simulink model "Parallel_R2017b"  (R2017b)
settings: Solver=ode4  StartTime=0  StopTime=1200  FixedStep=0.1  MaxStep=0.05  RelTol=1e-5
values from neighbouring files (symbols this model uses):
  Cd = 0.26    [Parallel_Initiate.m]
  Cr = 0.008    [Parallel_Initiate.m]
  Density = (85*19.6e6 + 15*32e6)/100    (= 21460000)    [Parallel_Initiate.m]
  Depletion = 0    [Parallel_Initiate.m]
  EMpower = EMpower_simulated(i)    [Batch_vary_rated_power.m]    (also in Parallel_Initiate.m = 50000)
  EtaICE = EtaICE_DIESEL    [Parallel_Initiate.m]
  EtaPE = 0.98    [Parallel_Initiate.m]
  grav = 9.81    [Parallel_Initiate.m]
  Hybrid = 1    [Parallel_Initiate.m]
  ICEpower = ICEpower_simulated(i)    [Batch_vary_rated_power.m]    (also in Parallel_Initiate.m = 65973)
  ksoc = max(Wbatt)/400/Tau_charge    [Parallel_Initiate.m]
  Mv = 1325 + 250    (= 1575)    [Parallel_Initiate.m]
  Number_of_gears = 5    [Parallel_Initiate.m]
  OnOffMax = SOC_batt_ref - eps    [Parallel_Initiate.m]
  OnOffMin = 30    [Parallel_Initiate.m]
  Paux = 600    [Parallel_Initiate.m]
  Pem_max = EMpower*Hybrid+2000*(1-Hybrid)    (= 50000)    [Parallel_Initiate.m]
  Pice_max = ICEpower*Hybrid+ICEconventional*(1-Hybrid)    (= 65973)    [Parallel_Initiate.m]
  rho_air = 1.225    [Parallel_Initiate.m]
  rw = 0.30    (= 0.3)    [Parallel_Initiate.m]
  SOC_batt_ref = 70    [Parallel_Initiate.m]
  StopAndGo = 0    [Parallel_Initiate.m]
  Tau_charge = 1    [Parallel_Initiate.m]
  Tem_max = TorqueEMmax*Hybrid+10*(1-Hybrid)    (= 400)    [Parallel_Initiate.m]
  Tice_max = Pice_max/(wice_max*row/(length(EtaICE)-1))    [Parallel_Initiate.m]
  utvx_max = wice_max/((vmax/5)/rw)    (= 15.9043128088)    [Parallel_Initiate.m]
  utvx_min = wice_max/(vmax/rw)/1.3    (= 2.4468173552)    [Parallel_Initiate.m]
  Utvx_vect = zeros(1,Number_of_gears+1)    [Parallel_Initiate.m]
  vmax = 160/3.6    (= 44.4444444444)    [Parallel_Initiate.m]
  Wbatt = 100*3600*13    (= 4680000)    [Parallel_Initiate.m]
  wice_max = 4500*2*pi/60    (= 471.238898038)    [Parallel_Initiate.m]
  wice_min = 800*2*pi/60    (= 83.7758040957)    [Parallel_Initiate.m]
undefined symbols (not defined in the file or in its folder): Av, EtaBATT, EtaEM, FuelConsICE, Pbatt, Pice_max_parallel, PtoT, sfunxy, Tem, Tice, Tlim_ice, Wem, Wice
libraries: simulink_need_slupdate x1
settings Model: ExtModeTrigMode=oneshot  ExtModeArmWhenConnect=off  Creator=matsl  LastModifiedBy=leksell
settings DataIOCC: SaveFormat=Array  SignalLoggingSaveFormat=ModelDataLogs  SignalLoggingName=sigsOut
settings OptimizationCC: BlockReduction=off  BooleanDataType=off  ExpressionDepthLimit=2147483647  InitFltsAndDblsToZero=on  LifeSpan=inf
settings DebuggingCC: ConsistencyChecking=warning  SaveWithParameterizedLinksMsg=none  UnderspecifiedInitializationDetection=Classic  MergeDetectMultiDrivingBlocksExec=none  SignalResolutionControl=TryResolveAllWithWarning  MultiTaskDSMMsg=warning  MultiTaskCondExecSysMsg=none  UnnecessaryDatatypeConvMsg=warning  FcnCallInpInsideContextMsg=warning  UnconnectedInputMsg=none  UnconnectedOutputMsg=none  UnconnectedLineMsg=none  AllowSymbolicDim=off  StateNameClashWarn=warning  SFUnexpectedBacktrackingDiag=warning  SFNoUnconditionalDefaultTransitionDiag=warning  SFExecutionAtInitializationDiag=none
settings HardwareCC: ProdBitPerPointer=32  ProdBitPerSizeT=32  ProdBitPerPtrDiffT=32  ProdLargestAtomicFloat=None  ProdIntDivRoundTo=Undefined  ProdEndianess=Unspecified  ProdWordSize=32  ProdHWDeviceType=32-bit Generic  TargetBitPerPointer=64  TargetBitPerSizeT=64  TargetBitPerPtrDiffT=64  TargetLongLongMode=on  TargetIntDivRoundTo=Zero  TargetEndianess=LittleEndian  TargetWordSize=64  TargetHWDeviceType=MATLAB Host  ProdEqTarget=off
settings ModelReferenceCC: PropagateSignalLabelsOutOfModel=off
settings CodeAppCC: StateflowObjectComments=on
settings GRTTargetCC: TargetFcnLib=ansi_tfl_tmw.mat  TargetLangStandard=C89/C90 (ANSI)  GeneratePreprocessorConditionals=Disable all  CombineOutputUpdateFcns=off  GRTInterface=on
settings ConfigComp: CovMetricSettings=dw  CovHtmlReporting=on  CovSaveCumulativeToWorkspaceVar=on  CovSaveSingleToWorkspaceVar=on  CovExternalEMLEnable=off

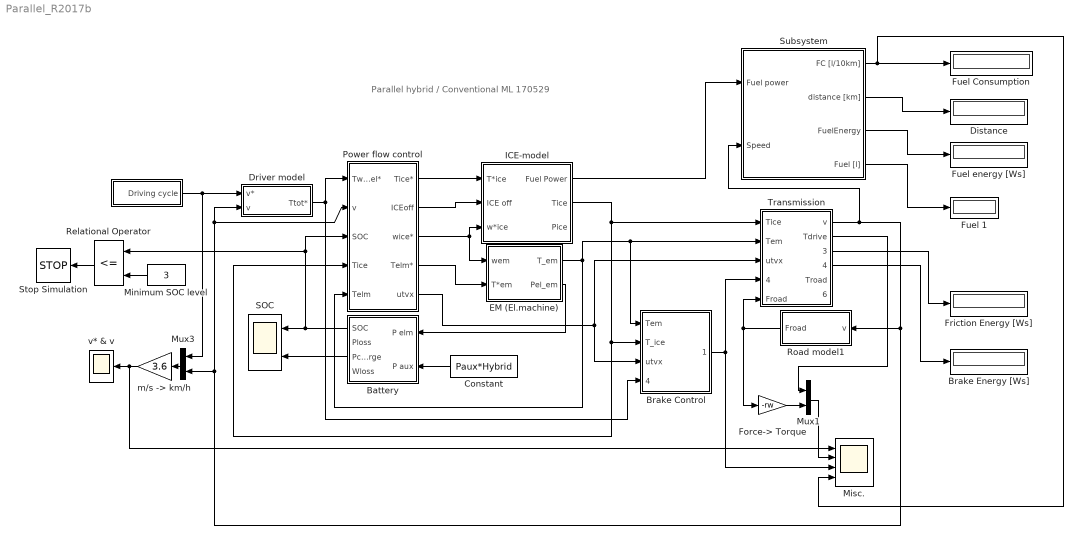
== system Parallel_R2017b ==
  note: Parallel hybrid / Conventional
      | ML 170529
  " " : Subsystem  mask{Cycle=us06}
      mask prompts: Cycle "Driving cycle"
      mask TypeOptions Cycle: nedc | us06 | IdealMotion
  Battery : Subsystem
  Brake Control : Subsystem
  Brake Energy [Ws] : Display
  Constant : Constant  Value=Paux*Hybrid
  Distance : Display
  "Driver model " : Subsystem  mask{Mv=Mv, rw=rw, T_max=(ICEpower+EMpower)/(vmax/rw)*utvx_min}
      mask prompts: Mv "Vehicle Mass"; rw "Wheel Radius"; T_max "Max Wheel Torque"
      mask init:
      | Ti = 3 + 7*(Mv-1000)/9000;
      | Kv=4*Mv/Ti;
  EM (El.machine) : Subsystem
  Force-> Torque : Gain  Gain=-rw  SaturateOnIntegerOverflow=on  OutDataTypeStr=Inherit: Same as input  ParamDataTypeStr=Inherit: Same as input
  Friction Energy [Ws] : Display
  Fuel 1 : Display
  Fuel Consumption : Display
  Fuel energy [Ws] : Display
  ICE-model : Subsystem
  Minimum SOC level : Constant  Value=3
  Misc. : Scope  NumInputPorts=4
  Mux1 : Mux  Inputs=2
  Mux3 : Mux  Inputs=2
  Power flow control : Subsystem
  Relational Operator : RelationalOperator  Operator=<=  OutDataTypeStr=boolean  RndMeth=Nearest
  Road model1 : Subsystem
  SOC : Scope  NumInputPorts=2
  Stop Simulation : Stop
  Subsystem : Subsystem
  Transmission : Subsystem
  "m/s -> km/h" : Gain  Gain=3.6  SaturateOnIntegerOverflow=on  OutDataTypeStr=Inherit: Same as input  ParamDataTypeStr=Inherit: Same as input
  v* & v : Scope
  wires:
  Power flow control/3(wice*) -> EM (El.machine)/1(wem), ICE-model/3(w*ice)
  Constant/1 -> Battery/2(P aux)
  " "/1(Driving cycle) -> Mux3/1, "Driver model "/1(v*)
  "Driver model "/1(Ttot*) -> Brake Control/4(T*_wheel), Power flow control/1(Twheel*)
  Mux3/1 -> "m/s -> km/h"/1
  Power flow control/5(utvx) -> Transmission/3(utvx), Brake Control/3(utvx)
  Power flow control/4(Telm*) -> EM (El.machine)/2(T*em)
  Power flow control/1(Tice*) -> ICE-model/1(T*ice)
  Transmission/1(v) -> "Driver model "/2(v), Power flow control/2(v), Mux3/2, Road model1/1("v "), Subsystem/2(Speed)
  Road model1/1(Froad) -> Transmission/5(Froad), Force-> Torque/1
  EM (El.machine)/1(T_em) -> Transmission/2(Tem), Brake Control/1(Tem), Power flow control/5(Telm)
  EM (El.machine)/2(Pel_em) -> Battery/1(P elm)
  "m/s -> km/h"/1 -> v* & v/1, Misc./1
  Transmission/3(Wfriction) -> Friction Energy [Ws]/1
  Transmission/4(Wbrake) -> Brake Energy [Ws]/1
  Subsystem/1(FC [l/10km]) -> Misc./4, Fuel Consumption/1
  Brake Control/1(T_brake) -> Transmission/4(Tbrake), Misc./3
  Power flow control/2(ICEoff) -> ICE-model/2(ICE off)
  Battery/3(Pcharge) -> SOC/2
  ICE-model/2(Tice) -> Transmission/1(Tice), Power flow control/4(Tice), Brake Control/2(T_ice)
  ICE-model/1(Fuel Power) -> Subsystem/1(Fuel power)
  Subsystem/3(FuelEnergy) -> Fuel energy [Ws]/1
  Force-> Torque/1 -> Mux1/2
  Mux1/1 -> Misc./2
  Transmission/2(Tdrive) -> Mux1/1
  Subsystem/2(distance [km]) -> Distance/1
  Subsystem/4(Fuel [l]) -> Fuel 1/1
  Relational Operator/1 -> Stop Simulation/1
  Minimum SOC level/1 -> Relational Operator/2
  Battery/1(SOC) -> Power flow control/3(SOC), Relational Operator/1, SOC/1

== system Parallel_R2017b/  ==
  Constant : Constant  Value=Cycle
  Multiport Switch : MultiPortSwitch  SaturateOnIntegerOverflow=on  InputSameDT=on
  v-buss1 : FromWorkspace  VariableName=us06  SampleTime=.1
  v-buss2 : FromWorkspace  VariableName=IdealMotion  SampleTime=.1
  v-buss8 : FromWorkspace  VariableName=nedc  SampleTime=.1
  Driving cycle : Outport
  wires:
  v-buss8/1 -> Multiport Switch/2
  Constant/1 -> Multiport Switch/1
  v-buss1/1 -> Multiport Switch/3
  v-buss2/1 -> Multiport Switch/4
  Multiport Switch/1 -> Driving cycle/1

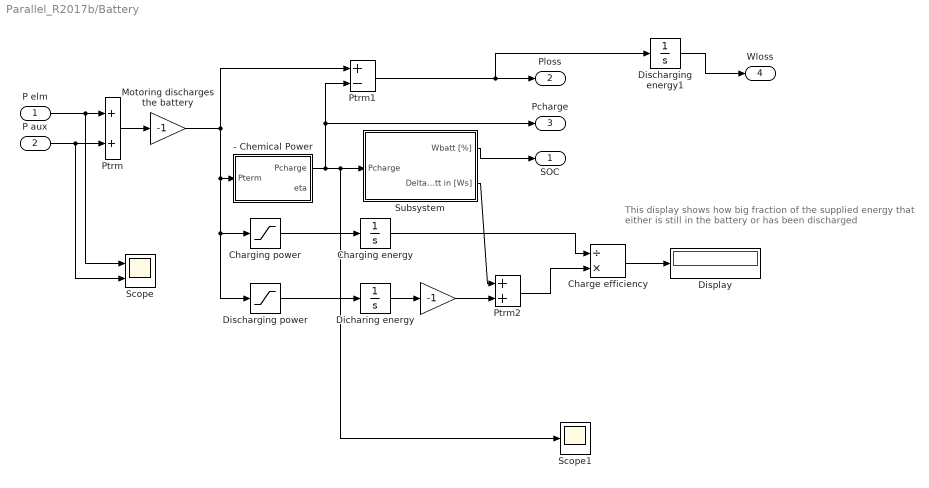
== system Parallel_R2017b/Battery ==
  note: This display shows how big fraction of the supplied energy
      | that either is still in the battery or has been discharged
  P elm : Inport
  P aux : Inport  Port=2
  " " : Gain  Gain=-1  SaturateOnIntegerOverflow=on  OutDataTypeStr=Inherit: Same as input  ParamDataTypeStr=Inherit: Same as input
  - Chemical Power : Subsystem
  Charge efficiency : Product  Inputs=/*  SaturateOnIntegerOverflow=on  OutDataTypeStr=Inherit: Same as first input
  Charging energy : Integrator  InitialCondition=1  LimitOutput=on  LowerSaturationLimit=1
  Charging power : Saturate  UpperLimit=inf  LowerLimit=0
  Dicharing energy : Integrator  InitialCondition=-1  LimitOutput=on  UpperSaturationLimit=-1
  Discharging energy1 : Integrator  UpperSaturationLimit=-1
  Discharging power : Saturate  UpperLimit=0  LowerLimit=-inf
  Display : Display
  Motoring discharges the battery : Gain  Gain=-1  SaturateOnIntegerOverflow=on  OutDataTypeStr=Inherit: Same as input  ParamDataTypeStr=Inherit: Same as input
  Ptrm : Sum  SaturateOnIntegerOverflow=on  InputSameDT=on  OutDataTypeStr=Inherit: Same as first input
  Ptrm1 : Sum  Inputs=+-  SaturateOnIntegerOverflow=on  InputSameDT=on  OutDataTypeStr=Inherit: Same as first input
  Ptrm2 : Sum  SaturateOnIntegerOverflow=on  InputSameDT=on  OutDataTypeStr=Inherit: Same as first input
  Scope : Scope  NumInputPorts=2
  Scope1 : Scope
  Subsystem : Subsystem
  SOC : Outport  InitialOutput=0
  Ploss : Outport  Port=2  InitialOutput=0
  Pcharge : Outport  Port=3  InitialOutput=0
  Wloss : Outport  Port=4  InitialOutput=0
  wires:
  P elm/1 -> Ptrm/1, Scope/1
  Ptrm/1 -> Motoring discharges the battery/1
  Subsystem/1(Wbatt [%]) -> SOC/1
  - Chemical Power/1(Pcharge) -> Ptrm1/2, Pcharge/1, Subsystem/1("Pcharge "), Scope1/1
  Ptrm1/1 -> Ploss/1, Discharging energy1/1
  Motoring discharges the battery/1 -> Ptrm1/1, Charging power/1, Discharging power/1, - Chemical Power/1(Pterm)
  Charge efficiency/1 -> Display/1
  Charging power/1 -> Charging energy/1
  Discharging power/1 -> Dicharing energy/1
  Dicharing energy/1 -> " "/1
  Subsystem/2(DeltaWbatt in [Ws]) -> Ptrm2/1
  " "/1 -> Ptrm2/2
  Ptrm2/1 -> Charge efficiency/2
  Charging energy/1 -> Charge efficiency/1
  P aux/1 -> Ptrm/2, Scope/2
  Discharging energy1/1 -> Wloss/1

== system Parallel_R2017b/Brake Control ==
  note: If the drive train is not able
      | to supply the braking force, then
      | the friction brakes are used.
  Tem : Inport
  T_ice : Inport  Port=2
  utvx : Inport  Port=3
  T*_wheel : Inport  Port=4
  -> wheel torque : Product  SaturateOnIntegerOverflow=on  InputSameDT=on  OutDataTypeStr=Inherit: Same as first input
  Only negative brake torque : Saturate  UpperLimit=0  LowerLimit=-inf
  Sum1 : Sum  Inputs=-+  SaturateOnIntegerOverflow=on  InputSameDT=on  OutDataTypeStr=Inherit: Same as first input
  Sum2 : Sum  SaturateOnIntegerOverflow=on  InputSameDT=on  OutDataTypeStr=Inherit: Same as first input
  T_brake : Outport  InitialOutput=0
  wires:
  Tem/1 -> Sum2/1
  T_ice/1 -> Sum2/2
  Sum2/1 -> -> wheel torque/1
  utvx/1 -> -> wheel torque/2
  -> wheel torque/1 -> Sum1/1
  T*_wheel/1 -> Sum1/2
  Sum1/1 -> Only negative brake torque/1
  Only negative brake torque/1 -> T_brake/1

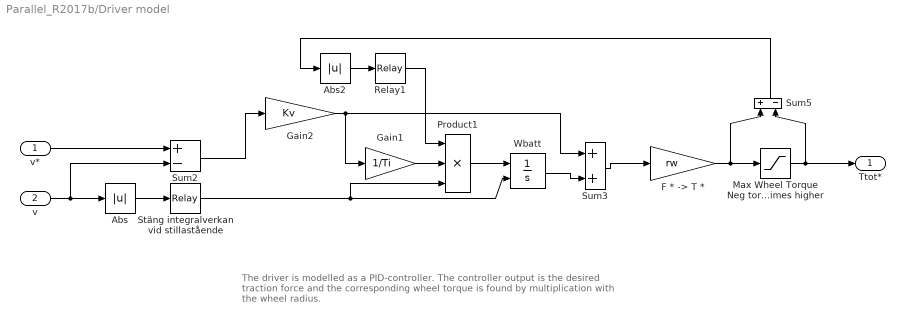
== system Parallel_R2017b/Driver model  ==
  note: The driver is modelled as a PID-controller.
      | The controller output is the desired traction force and the
      | corresponding wheel torque is found by multiplication with the wheel radius.
  v* : Inport
  v : Inport  Port=2
  Abs : Abs  SaturateOnIntegerOverflow=on
  Abs2 : Abs  SaturateOnIntegerOverflow=on
  "F * -> T *" : Gain  Gain=rw  SaturateOnIntegerOverflow=on  OutDataTypeStr=Inherit: Same as input  ParamDataTypeStr=Inherit: Same as input
  Gain1 : Gain  Gain=1/Ti  SaturateOnIntegerOverflow=on  OutDataTypeStr=Inherit: Same as input  ParamDataTypeStr=Inherit: Same as input
  Gain2 : Gain  Gain=Kv  SaturateOnIntegerOverflow=on  OutDataTypeStr=Inherit: Same as input  ParamDataTypeStr=Inherit: Same as input
  Max Wheel Torque Neg torque 5 times higher : Saturate  UpperLimit=T_max  LowerLimit=-T_max*5
  Product1 : Product  Inputs=3  SaturateOnIntegerOverflow=on  InputSameDT=on  OutDataTypeStr=Inherit: Same as first input
  Relay1 : Relay  OnOutputValue=0  OffOutputValue=1
  Stäng integralverkan vid stillastående : Relay  OnSwitchValue=0.3  OffSwitchValue=0.3-eps
  Sum2 : Sum  Inputs=+-  SaturateOnIntegerOverflow=on  InputSameDT=on  OutDataTypeStr=Inherit: Same as first input
  Sum3 : Sum  SaturateOnIntegerOverflow=on  InputSameDT=on  OutDataTypeStr=Inherit: Same as first input
  Sum5 : Sum  Inputs=+-  SaturateOnIntegerOverflow=on  InputSameDT=on  OutDataTypeStr=Inherit: Same as first input
  Wbatt : Integrator  ExternalReset=falling  LimitOutput=on  UpperSaturationLimit=1000  LowerSaturationLimit=-10000
  Ttot* : Outport  InitialOutput=0
  wires:
  Sum5/1 -> Abs2/1
  Max Wheel Torque Neg torque 5 times higher/1 -> Sum5/2, Ttot*/1
  Relay1/1 -> Product1/1
  Abs2/1 -> Relay1/1
  Gain1/1 -> Product1/2
  Abs/1 -> Stäng integralverkan vid stillastående/1
  Product1/1 -> Wbatt/1
  Sum3/1 -> "F * -> T *"/1
  Wbatt/1 -> Sum3/2
  "F * -> T *"/1 -> Sum5/1, Max Wheel Torque Neg torque 5 times higher/1
  Gain2/1 -> Gain1/1, Sum3/1
  Stäng integralverkan vid stillastående/1 -> Product1/3, Wbatt/2
  Sum2/1 -> Gain2/1
  v*/1 -> Sum2/1
  v/1 -> Abs/1, Sum2/2

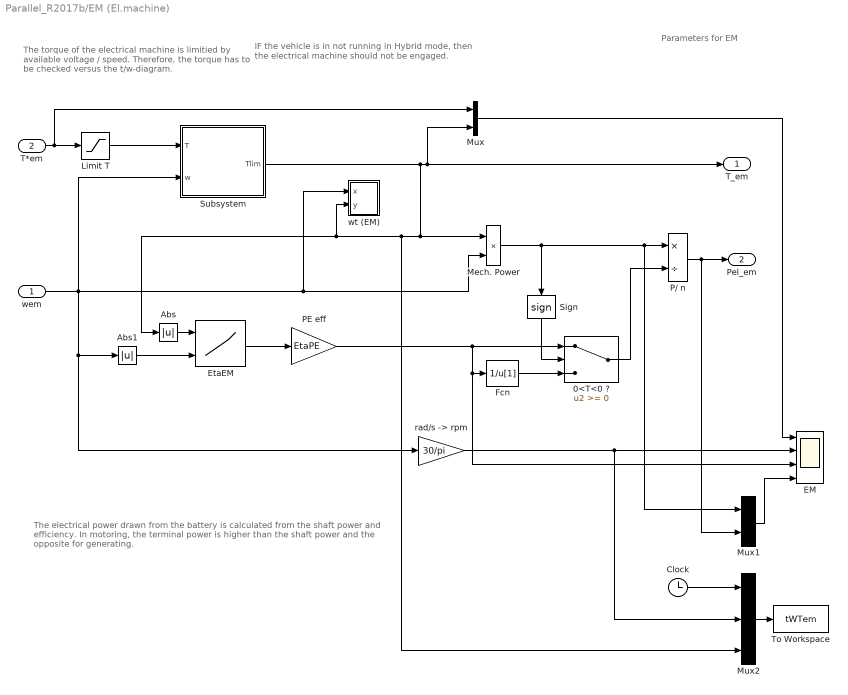
== system Parallel_R2017b/EM (El.machine) ==
  note: The torque of the electrical machine is
      | limitied by available voltage / speed. Therefore, the
      | torque has to be checked versus the t/w-diagram.
  note: IF the vehicle is in not running in Hybrid mode, then
      | the electrical machine should not be engaged.
  note: The electrical power drawn from the battery is calculated from the shaft power and
      | efficiency. In motoring, the terminal power is higher than the shaft power and
      | the opposite for  generating.
  note: Parameters for EM
  wem : Inport
  T*em : Inport  Port=2
  0<T<0 ? : Switch  SaturateOnIntegerOverflow=on  InputSameDT=on
  Abs : Abs  SaturateOnIntegerOverflow=on
  Abs1 : Abs  SaturateOnIntegerOverflow=on
  Clock : Clock
  "EM " : Scope  NumInputPorts=4
  EtaEM : Lookup2D  RowIndex=Tem  ColumnIndex=Wem  Table=EtaEM  LookUpMeth=Interpolation-Use End Values  SaturateOnIntegerOverflow=on
  Fcn : Fcn  Expr=1/u[1]
  Limit T : Saturate  UpperLimit=Tem_max  LowerLimit=-Tem_max
  Mech. Power : Product  SaturateOnIntegerOverflow=on  OutDataTypeStr=Inherit: Same as first input
  Mux : Mux  Inputs=2
  Mux1 : Mux  Inputs=2
  Mux2 : Mux  Inputs=3
  P/ n : Product  Inputs=*/  SaturateOnIntegerOverflow=on  InputSameDT=on  OutDataTypeStr=Inherit: Same as first input
  PE eff : Gain  Gain=EtaPE  SaturateOnIntegerOverflow=on  OutDataTypeStr=Inherit: Same as input  ParamDataTypeStr=Inherit: Same as input
  Sign : Signum
  Subsystem : Subsystem  mask{Tmax=Tem_max, Pmax=Pem_max}
      mask prompts: Tmax "Max Torque"; Pmax "Max Power"
      mask Display:
      | plot(-120,-120,120,120)
      | plot([-110 110],[0 0],[0 0],[-110 110])
      | plot([-20 20],[90 90],[-20 20],[-90 -90])
      | 
      | plot([-100 :-20],-90*20./[-100:-20])
      | plot([-100 :-20],90*20./[-100:-20])
      | plot([20:100],-90*20./[20:100])
      | plot([20:100],90*20./[20:100])
  To Workspace : ToWorkspace  VariableName=tWTem  SampleTime=-1
  "rad/s -> rpm" : Gain  Gain=30/pi  SaturateOnIntegerOverflow=on  OutDataTypeStr=Inherit: Same as input  ParamDataTypeStr=Inherit: Same as input
  wt (EM) : Subsystem  AncestorBlock=simulink/Sinks/XY Graph  LoadFcn=sfunxy([],[],[],'LoadBlock')  StartFcn=sfunxy([],[],[],'Start')  StopFcn=sfunxy([],[],[],'Stop')  TreatAsAtomicUnit=on  SimViewingDevice=on  mask(XY scope.){xmin=-max(Wem)*1.2, xmax=max(Wem)*1.2, ymin=-max(Tem)*1.2, ymax=max(Tem)*1.2, st=1}
      mask prompts: xmin "x-min:"; xmax "x-max:"; ymin "y-min:"; ymax "y-max:"; st "Sample time:"
      mask help: Plots second input (Y) against first input (X) at each time step to create an X-Y plot. Ignores data outside the ranges specified by x-min, x-max, y-min, y-max.
      settings: CopyFcn=sfunxy([],[],[],'CopyBlock')  DeleteFcn=sfunxy([],[],[],'DeleteBlock')  NameChangeFcn=sfunxy([],[],[],'NameChange')
      mask Help: This block can be used to explore limit cycles. Look at the m-file sfunxy.m to see how it works.
      mask Display: plot([.05 .95 .95 .05 .05],[.45 .45 .95 .95 .45], 0.5+cos(0:0.1:2*pi)*0.3,0.7+sin(0:0.1:2*pi)*0.2)
  T_em : Outport  InitialOutput=0
  Pel_em : Outport  Port=2  InitialOutput=0
  wires:
  EtaEM/1 -> PE eff/1
  Sign/1 -> 0<T<0 ?/2
  P/ n/1 -> Mux1/2, Pel_em/1
  T*em/1 -> Limit T/1, Mux/1
  Fcn/1 -> 0<T<0 ?/3
  0<T<0 ?/1 -> P/ n/2
  Abs/1 -> EtaEM/1
  Limit T/1 -> Subsystem/1(T)
  PE eff/1 -> "EM "/3, Fcn/1, 0<T<0 ?/1
  Mux/1 -> "EM "/1
  Mux1/1 -> "EM "/4
  Mech. Power/1 -> Sign/1, Mux1/1, P/ n/1
  Abs1/1 -> EtaEM/2
  wem/1 -> "rad/s -> rpm"/1, Abs1/1, wt (EM)/1(x), Mech. Power/2, Subsystem/2(w)
  Subsystem/1(Tlim) -> T_em/1, Mux/2, Mech. Power/1, wt (EM)/2(y), Abs/1, Mux2/3
  Clock/1 -> Mux2/1
  Mux2/1 -> To Workspace/1
  "rad/s -> rpm"/1 -> Mux2/2, "EM "/2

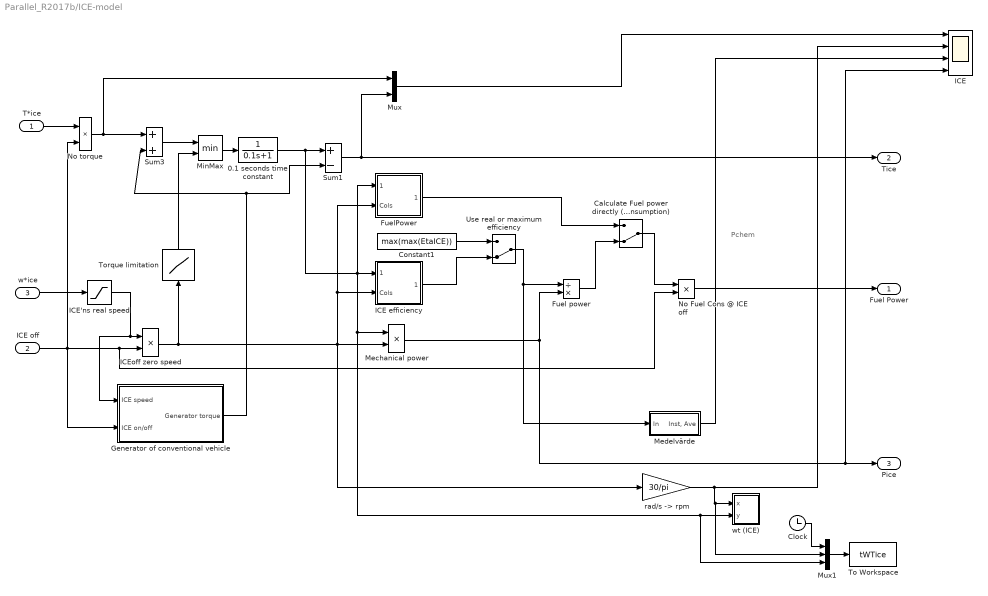
== system Parallel_R2017b/ICE-model ==
  note: Pchem
  T*ice : Inport
  ICE off : Inport  Port=2
  w*ice : Inport  Port=3
  0.1 seconds time constant : TransferFcn  Denominator=[0.1 1]
  Calculate Fuel power directly (w/o idle consumption) : ManualSwitch  CurrentSetting=0
  Clock : Clock
  Constant1 : Constant  Value=max(max(EtaICE))
  Fuel power : Product  Inputs=/*  SaturateOnIntegerOverflow=on  InputSameDT=on  OutDataTypeStr=Inherit: Same as first input
  FuelPower : Subsystem  mask(Lookup Table (2-D)){x=Tice, y=Wice, t=FuelConsICE}
      mask prompts: x "Row:"; y "Column:"; t "Table:"
      mask help: Performs 2-D linear interpolation of input values using the specified input/output table. Extrapolation is performed outside the table boundaries. The first dimension corresponds to the top (or left) input port.
      mask init:
      | [r,c]=size(t);
      | xt=reshape(x,prod(size(x)),1);
      | xi=xt(:,ones(1,c));
      | minx=min(x); maxx=max(x);
      | mint=min(min(t)); maxt=max(max(t));
      mask Display: plot(double(xi),double(t),double([minx maxx]),double([mint mint]),double([minx minx]),double([mint maxt]))
  Generator of conventional vehicle : Subsystem
  ICE : Scope  NumInputPorts=4
  ICE efficiency : Subsystem  mask(Lookup Table (2-D)){x=Tice, y=Wice, t=EtaICE}
      mask prompts: x "Row:"; y "Column:"; t "Table:"
      mask help: Performs 2-D linear interpolation of input values using the specified input/output table. Extrapolation is performed outside the table boundaries. The first dimension corresponds to the top (or left) input port.
      mask init:
      | [r,c]=size(t);
      | xt=reshape(x,prod(size(x)),1);
      | xi=xt(:,ones(1,c));
      | minx=min(x); maxx=max(x);
      | mint=min(min(t)); maxt=max(max(t));
      mask Display: plot(double(xi),double(t),double([minx maxx]),double([mint mint]),double([minx minx]),double([mint maxt]))
  ICE'ns real speed : Saturate  UpperLimit=wice_max  LowerLimit=wice_min
  ICEoff zero speed : Product  SaturateOnIntegerOverflow=on  InputSameDT=on  OutDataTypeStr=Inherit: Same as first input
  Mechanical power : Product  SaturateOnIntegerOverflow=on  InputSameDT=on  OutDataTypeStr=Inherit: Same as first input
  Medelvärde : Subsystem
  MinMax : MinMax  Inputs=2  SaturateOnIntegerOverflow=on  InputSameDT=on
  Mux : Mux  Inputs=2
  Mux1 : Mux  Inputs=3
  No Fuel Cons @ ICE off : Product  Inputs=**  SaturateOnIntegerOverflow=on  InputSameDT=on  OutDataTypeStr=Inherit: Same as first input
  No torque : Product  SaturateOnIntegerOverflow=on  OutDataTypeStr=Inherit: Same as first input
  Sum1 : Sum  Inputs=+-  SaturateOnIntegerOverflow=on
  Sum3 : Sum  SaturateOnIntegerOverflow=on
  To Workspace : ToWorkspace  VariableName=tWTice  SampleTime=-1
  Torque limitation : Lookup  InputValues=Wice  Table=Tlim_ice  SaturateOnIntegerOverflow=on
  Use real or maximum efficiency : ManualSwitch  CurrentSetting=0
  "rad/s -> rpm" : Gain  Gain=30/pi  SaturateOnIntegerOverflow=on  OutDataTypeStr=Inherit: Same as input  ParamDataTypeStr=Inherit: Same as input
  wt (ICE) : Subsystem  AncestorBlock=simulink/Sinks/XY Graph  LoadFcn=sfunxy([],[],[],'LoadBlock')  StartFcn=sfunxy([],[],[],'Start')  StopFcn=sfunxy([],[],[],'Stop')  TreatAsAtomicUnit=on  SimViewingDevice=on  mask(XY scope.){xmin=0, xmax=max(Wice)*30/pi*1.2, ymin=-max(Tice)*0.2, ymax=max(Tice)*1.2, st=1}
      mask prompts: xmin "x-min:"; xmax "x-max:"; ymin "y-min:"; ymax "y-max:"; st "Sample time:"
      mask help: Plots second input (Y) against first input (X) at each time step to create an X-Y plot. Ignores data outside the ranges specified by x-min, x-max, y-min, y-max.
      settings: CopyFcn=sfunxy([],[],[],'CopyBlock')  DeleteFcn=sfunxy([],[],[],'DeleteBlock')  NameChangeFcn=sfunxy([],[],[],'NameChange')
      mask Help: This block can be used to explore limit cycles. Look at the m-file sfunxy.m to see how it works.
      mask Display: plot([.05 .95 .95 .05 .05],[.45 .45 .95 .95 .45], 0.5+cos(0:0.1:2*pi)*0.3,0.7+sin(0:0.1:2*pi)*0.2)
  Fuel Power : Outport  InitialOutput=0
  Tice : Outport  Port=2  InitialOutput=0
  Pice : Outport  Port=3  InitialOutput=0
  wires:
  Mux/1 -> ICE/1
  MinMax/1 -> 0.1 seconds time constant/1
  Torque limitation/1 -> MinMax/2
  Medelvärde/1("Inst, Ave") -> ICE/3
  w*ice/1 -> ICE'ns real speed/1
  No torque/1 -> Sum3/1, Mux/1
  Mechanical power/1 -> Fuel power/2, Pice/1, ICE/4
  Generator of conventional vehicle/1(Generator torque) -> Sum3/2, Sum1/2
  Sum1/1 -> Tice/1, Mux/2
  Sum3/1 -> MinMax/1
  ICE off/1 -> Generator of conventional vehicle/2(ICE on/off), ICEoff zero speed/2, No Fuel Cons @ ICE off/2, No torque/2
  Fuel power/1 -> Calculate Fuel power directly (w/o idle consumption)/2
  Calculate Fuel power directly (w/o idle consumption)/1 -> No Fuel Cons @ ICE off/1
  No Fuel Cons @ ICE off/1 -> Fuel Power/1
  FuelPower/1(Out1) -> Calculate Fuel power directly (w/o idle consumption)/1
  Constant1/1 -> Use real or maximum efficiency/1
  ICE efficiency/1(Out1) -> Use real or maximum efficiency/2
  Use real or maximum efficiency/1 -> Fuel power/1, Medelvärde/1(In)
  ICE'ns real speed/1 -> Generator of conventional vehicle/1(ICE speed), ICEoff zero speed/1
  ICEoff zero speed/1 -> Torque limitation/1, FuelPower/2(Cols), ICE efficiency/2(Cols), Mechanical power/2, "rad/s -> rpm"/1
  T*ice/1 -> No torque/1
  "rad/s -> rpm"/1 -> Mux1/2, wt (ICE)/1(x), ICE/2
  Clock/1 -> Mux1/1
  Mux1/1 -> To Workspace/1
  0.1 seconds time constant/1 -> Sum1/1, ICE efficiency/1(Rows), Mechanical power/1, Mux1/3, wt (ICE)/2(y), FuelPower/1(Rows)

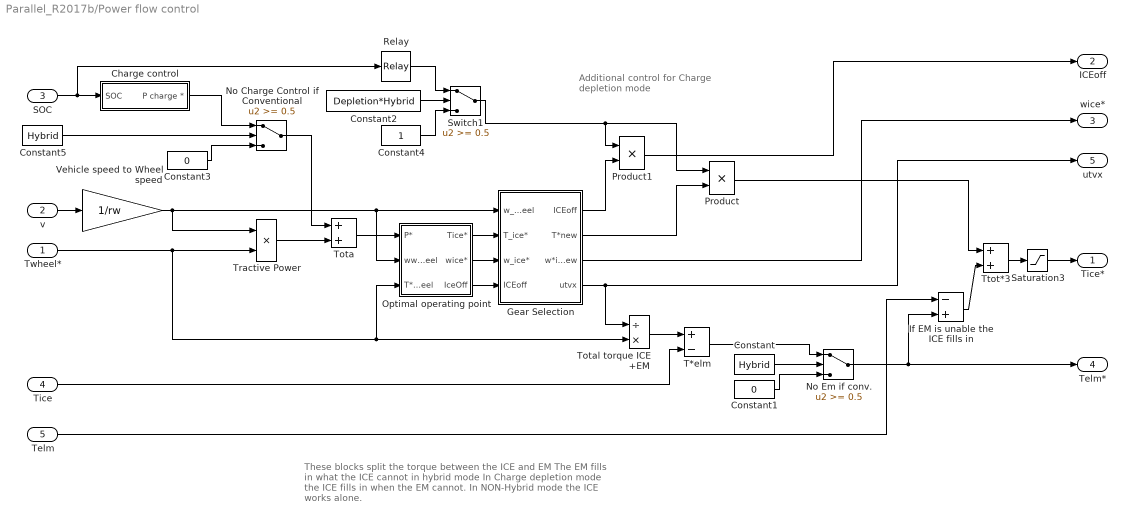
== system Parallel_R2017b/Power flow control ==
  note: Additional control for
      | Charge depletion mode
  note: These blocks split the torque between the ICE and EM
      | The EM fills in what the ICE cannot in hybrid mode
      |
      | In Charge depletion mode the ICE fills in when the EM cannot.
      |
      | In NON-Hybrid mode the ICE works alone.
  Twheel* : Inport
  v : Inport  Port=2
  SOC : Inport  Port=3
  Tice : Inport  Port=4
  Telm : Inport  Port=5
  Charge control : Subsystem
  Constant : Constant  Value=Hybrid
  Constant1 : Constant  Value=0
  Constant2 : Constant  Value=Depletion*Hybrid
  Constant3 : Constant  Value=0
  Constant4 : Constant
  Constant5 : Constant  Value=Hybrid
  Gear Selection : Subsystem
  If EM is unable the ICE fills in : Sum  Inputs=-+  SaturateOnIntegerOverflow=on  InputSameDT=on  OutDataTypeStr=Inherit: Same as first input
  No Charge Control if Conventional : Switch  Threshold=0.5  SaturateOnIntegerOverflow=on  InputSameDT=on
  No Em if conv. : Switch  Threshold=0.5  SaturateOnIntegerOverflow=on  InputSameDT=on
  Optimal operating point : Subsystem
  Product : Product  SaturateOnIntegerOverflow=on  OutDataTypeStr=Inherit: Same as first input
  Product1 : Product  SaturateOnIntegerOverflow=on  OutDataTypeStr=Inherit: Same as first input
  Relay : Relay  OnSwitchValue=OnOffMax  OffSwitchValue=OnOffMin  OnOutputValue=0  OffOutputValue=1
  Saturation3 : Saturate  UpperLimit=Tice_max  LowerLimit=eps
  Switch1 : Switch  Threshold=0.5  SaturateOnIntegerOverflow=on  InputSameDT=on
  T*elm : Sum  Inputs=+-  SaturateOnIntegerOverflow=on  InputSameDT=on  OutDataTypeStr=Inherit: Same as first input
  Tota : Sum  SaturateOnIntegerOverflow=on  InputSameDT=on  OutDataTypeStr=Inherit: Same as first input
  Total torque ICE +EM : Product  Inputs=/*  SaturateOnIntegerOverflow=on  InputSameDT=on  OutDataTypeStr=Inherit: Same as first input
  Tractive Power : Product  SaturateOnIntegerOverflow=on  InputSameDT=on  OutDataTypeStr=Inherit: Same as first input
  Ttot*3 : Sum  SaturateOnIntegerOverflow=on  InputSameDT=on  OutDataTypeStr=Inherit: Same as first input
  Vehicle speed to Wheel speed : Gain  Gain=1/rw  SaturateOnIntegerOverflow=on  OutDataTypeStr=Inherit: Same as input  ParamDataTypeStr=Inherit: Same as input
  Tice* : Outport
  ICEoff : Outport  Port=2
  wice* : Outport  Port=3
  Telm* : Outport  Port=4
  utvx : Outport  Port=5
  wires:
  Vehicle speed to Wheel speed/1 -> Tractive Power/1, Gear Selection/1(w_wheel), Optimal operating point/2(wwheel)
  Twheel*/1 -> Tractive Power/2, Total torque ICE +EM/2, Optimal operating point/3(T*wheel)
  v/1 -> Vehicle speed to Wheel speed/1
  Gear Selection/4(utvx) -> Total torque ICE +EM/1, utvx/1
  Optimal operating point/2(wice*) -> Gear Selection/3(w_ice*)
  Optimal operating point/1(Tice*) -> Gear Selection/2(T_ice*)
  SOC/1 -> Charge control/1(SOC), Relay/1
  Tractive Power/1 -> Tota/2
  Tota/1 -> Optimal operating point/1(P*)
  Gear Selection/3(w*ice_new) -> wice*/1
  Constant/1 -> No Em if conv./2
  Charge control/1(P charge *) -> No Charge Control if Conventional/1
  T*elm/1 -> No Em if conv./1
  No Em if conv./1 -> Telm*/1, If EM is unable the ICE fills in/2
  Constant1/1 -> No Em if conv./3
  No Charge Control if Conventional/1 -> Tota/1
  Constant3/1 -> No Charge Control if Conventional/3
  Tice/1 -> T*elm/2
  Total torque ICE +EM/1 -> T*elm/1
  Constant4/1 -> Switch1/3
  Relay/1 -> Switch1/1
  Telm/1 -> If EM is unable the ICE fills in/1
  If EM is unable the ICE fills in/1 -> Ttot*3/2
  Saturation3/1 -> Tice*/1
  Ttot*3/1 -> Saturation3/1
  Gear Selection/2(T*new) -> Product/2
  Product/1 -> Ttot*3/1
  Constant2/1 -> Switch1/2
  Constant5/1 -> No Charge Control if Conventional/2
  Product1/1 -> ICEoff/1
  Gear Selection/1("ICEoff ") -> Product1/2
  Switch1/1 -> Product/1, Product1/1
  Optimal operating point/3(IceOff) -> Gear Selection/4(ICEoff)

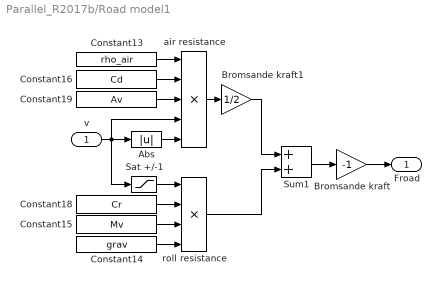
== system Parallel_R2017b/Road model1 ==
  "v " : Inport
  Abs : Abs  SaturateOnIntegerOverflow=on
  Bromsande kraft : Gain  Gain=-1  SaturateOnIntegerOverflow=on  OutDataTypeStr=Inherit: Same as input  ParamDataTypeStr=Inherit: Same as input
  Bromsande kraft1 : Gain  Gain=1/2  SaturateOnIntegerOverflow=on  OutDataTypeStr=Inherit: Same as input  ParamDataTypeStr=Inherit: Same as input
  Constant13 : Constant  Value=rho_air
  Constant14 : Constant  Value=grav
  Constant15 : Constant  Value=Mv
  Constant16 : Constant  Value=Cd
  Constant18 : Constant  Value=Cr
  Constant19 : Constant  Value=Av
  Sat +/-1 : Saturate  UpperLimit=1  LowerLimit=-1
  Sum1 : Sum  SaturateOnIntegerOverflow=on  InputSameDT=on  OutDataTypeStr=Inherit: Same as first input
  air resistance : Product  Inputs=5  SaturateOnIntegerOverflow=on  InputSameDT=on  OutDataTypeStr=Inherit: Same as first input
  roll resistance : Product  Inputs=4  SaturateOnIntegerOverflow=on  InputSameDT=on  OutDataTypeStr=Inherit: Same as first input
  Froad : Outport  InitialOutput=0
  wires:
  Abs/1 -> air resistance/5
  Sat +/-1/1 -> roll resistance/1
  Constant14/1 -> roll resistance/4
  Constant15/1 -> roll resistance/3
  Constant18/1 -> roll resistance/2
  "v "/1 -> Abs/1, Sat +/-1/1, air resistance/4
  Constant19/1 -> air resistance/3
  Constant16/1 -> air resistance/2
  Constant13/1 -> air resistance/1
  Sum1/1 -> Bromsande kraft/1
  roll resistance/1 -> Sum1/2
  Bromsande kraft1/1 -> Sum1/1
  Bromsande kraft/1 -> Froad/1
  air resistance/1 -> Bromsande kraft1/1

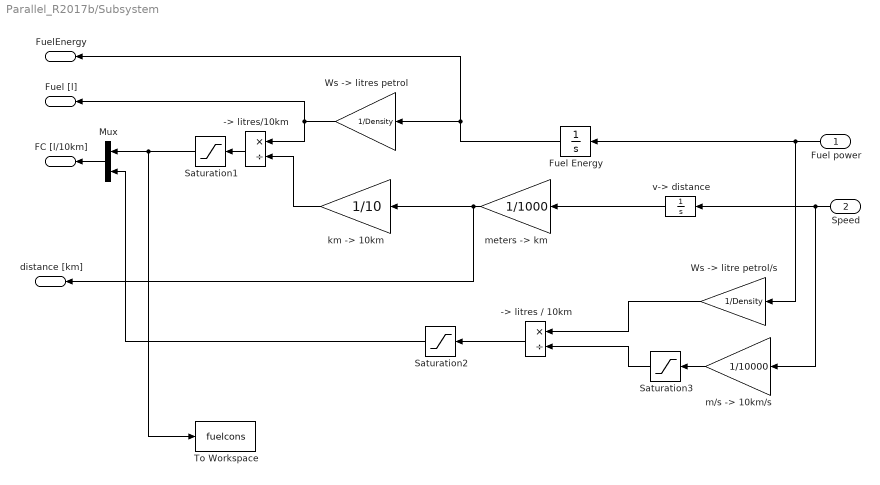
== system Parallel_R2017b/Subsystem ==
  Fuel power : Inport
  Speed : Inport  Port=2
  -> litres / 10km : Product  Inputs=*/  SaturateOnIntegerOverflow=on  InputSameDT=on  OutDataTypeStr=Inherit: Same as first input
  -> litres/10km : Product  Inputs=*/  SaturateOnIntegerOverflow=on  InputSameDT=on  OutDataTypeStr=Inherit: Same as first input
  Fuel Energy : Integrator
  Mux : Mux  Inputs=2
  Saturation1 : Saturate  UpperLimit=5  LowerLimit=eps
  Saturation2 : Saturate  UpperLimit=5  LowerLimit=eps
  Saturation3 : Saturate  UpperLimit=inf  LowerLimit=eps
  To Workspace : ToWorkspace  VariableName=fuelcons  SampleTime=-1
  "Ws -> litre petrol/s" : Gain  Gain=1/Density  SaturateOnIntegerOverflow=on  OutDataTypeStr=Inherit: Same as input  ParamDataTypeStr=Inherit: Same as input
  "Ws -> litres petrol" : Gain  Gain=1/Density  SaturateOnIntegerOverflow=on  OutDataTypeStr=Inherit: Same as input  ParamDataTypeStr=Inherit: Same as input
  "km -> 10km" : Gain  Gain=1/10  SaturateOnIntegerOverflow=on  OutDataTypeStr=Inherit: Same as input  ParamDataTypeStr=Inherit: Same as input
  "m/s -> 10km/s" : Gain  Gain=1/10000  SaturateOnIntegerOverflow=on  OutDataTypeStr=Inherit: Same as input  ParamDataTypeStr=Inherit: Same as input
  "meters -> km" : Gain  Gain=1/1000  SaturateOnIntegerOverflow=on  OutDataTypeStr=Inherit: Same as input  ParamDataTypeStr=Inherit: Same as input
  v-> distance : Integrator  InitialCondition=100  LimitOutput=on  LowerSaturationLimit=100
  FC [l/10km] : Outport
  distance [km] : Outport  Port=2
  FuelEnergy : Outport  Port=3
  Fuel [l] : Outport  Port=4
  wires:
  "Ws -> litres petrol"/1 -> -> litres/10km/1, Fuel [l]/1
  v-> distance/1 -> "meters -> km"/1
  -> litres/10km/1 -> Saturation1/1
  Speed/1 -> v-> distance/1, "m/s -> 10km/s"/1
  "meters -> km"/1 -> distance [km]/1, "km -> 10km"/1
  Fuel Energy/1 -> "Ws -> litres petrol"/1, FuelEnergy/1
  Fuel power/1 -> Fuel Energy/1, "Ws -> litre petrol/s"/1
  -> litres / 10km/1 -> Saturation2/1
  "Ws -> litre petrol/s"/1 -> -> litres / 10km/1
  "m/s -> 10km/s"/1 -> Saturation3/1
  Saturation1/1 -> To Workspace/1, Mux/1
  Mux/1 -> FC [l/10km]/1
  Saturation3/1 -> -> litres / 10km/2
  Saturation2/1 -> Mux/2
  "km -> 10km"/1 -> -> litres/10km/2

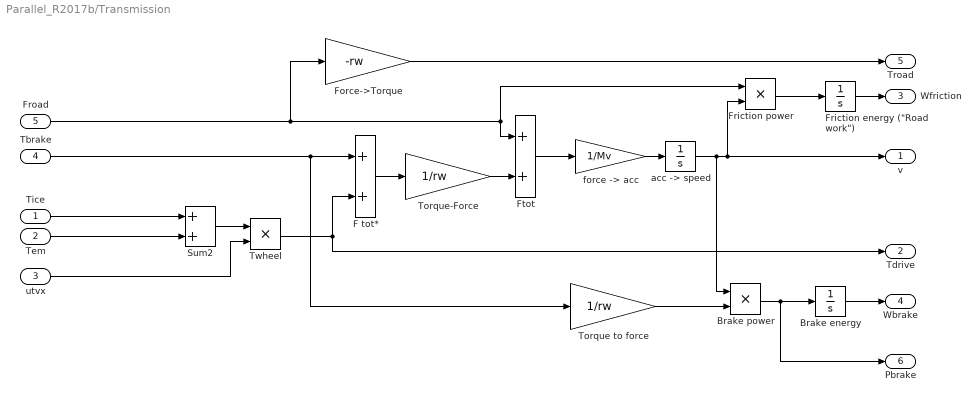
== system Parallel_R2017b/Transmission ==
  Tice : Inport
  Tem : Inport  Port=2
  utvx : Inport  Port=3
  Tbrake : Inport  Port=4
  Froad : Inport  Port=5
  Brake energy : Integrator
  Brake power : Product  SaturateOnIntegerOverflow=on  InputSameDT=on  OutDataTypeStr=Inherit: Same as first input
  F tot* : Sum  SaturateOnIntegerOverflow=on  InputSameDT=on  OutDataTypeStr=Inherit: Same as first input
  Force->Torque : Gain  Gain=-rw  SaturateOnIntegerOverflow=on  OutDataTypeStr=Inherit: Same as input  ParamDataTypeStr=Inherit: Same as input
  "Friction energy (\"Road work\")" : Integrator
  Friction power : Product  SaturateOnIntegerOverflow=on  InputSameDT=on  OutDataTypeStr=Inherit: Same as first input
  Ftot : Sum  SaturateOnIntegerOverflow=on  InputSameDT=on  OutDataTypeStr=Inherit: Same as first input
  Sum2 : Sum  SaturateOnIntegerOverflow=on  InputSameDT=on  OutDataTypeStr=Inherit: Same as first input
  Torque to force : Gain  Gain=1/rw  SaturateOnIntegerOverflow=on  OutDataTypeStr=Inherit: Same as input  ParamDataTypeStr=Inherit: Same as input
  Torque-Force : Gain  Gain=1/rw  SaturateOnIntegerOverflow=on  OutDataTypeStr=Inherit: Same as input  ParamDataTypeStr=Inherit: Same as input
  Twheel : Product  SaturateOnIntegerOverflow=on  InputSameDT=on  OutDataTypeStr=Inherit: Same as first input
  "acc -> speed" : Integrator  LimitOutput=on  LowerSaturationLimit=0
  "force -> acc" : Gain  Gain=1/Mv  SaturateOnIntegerOverflow=on  OutDataTypeStr=Inherit: Same as input  ParamDataTypeStr=Inherit: Same as input
  v : Outport  InitialOutput=0
  Tdrive : Outport  Port=2  InitialOutput=0
  Wfriction : Outport  Port=3  InitialOutput=0
  Wbrake : Outport  Port=4  InitialOutput=0
  Troad : Outport  Port=5  InitialOutput=0
  Pbrake : Outport  Port=6  InitialOutput=0
  wires:
  "force -> acc"/1 -> "acc -> speed"/1
  Tice/1 -> Sum2/1
  Tem/1 -> Sum2/2
  "acc -> speed"/1 -> v/1, Friction power/2, Brake power/1
  Sum2/1 -> Twheel/1
  utvx/1 -> Twheel/2
  F tot*/1 -> Torque-Force/1
  Twheel/1 -> F tot*/2, Tdrive/1
  Tbrake/1 -> F tot*/1, Torque to force/1
  Torque-Force/1 -> Ftot/2
  Ftot/1 -> "force -> acc"/1
  Froad/1 -> Ftot/1, Friction power/1, Force->Torque/1
  Torque to force/1 -> Brake power/2
  Brake power/1 -> Brake energy/1, Pbrake/1
  Friction power/1 -> "Friction energy (\"Road work\")"/1
  "Friction energy (\"Road work\")"/1 -> Wfriction/1
  Brake energy/1 -> Wbrake/1
  Force->Torque/1 -> Troad/1

== system Parallel_R2017b/Battery/- Chemical Power ==
  Pterm : Inport
  Look-Up Table : Lookup  InputValues=Pbatt  Table=EtaBATT  LookUpMeth=Interpolation-Use End Values  SaturateOnIntegerOverflow=on
  P/ n : Product  Inputs=**  SaturateOnIntegerOverflow=on  InputSameDT=on  OutDataTypeStr=Inherit: Same as first input
  Saturation : Saturate  UpperLimit=max(Pbatt)  LowerLimit=min(Pbatt)
  Pcharge : Outport  InitialOutput=0
  eta : Outport  Port=2  InitialOutput=0
  wires:
  Pterm/1 -> P/ n/1, Saturation/1
  Saturation/1 -> Look-Up Table/1
  P/ n/1 -> Pcharge/1
  Look-Up Table/1 -> P/ n/2, eta/1

== system Parallel_R2017b/Battery/Subsystem ==
  "Pcharge " : Inport
  Constant : Constant  Value=Wbatt*SOC_batt_ref/100
  Gain3 : Gain  Gain=100/Wbatt  SaturateOnIntegerOverflow=on  OutDataTypeStr=Inherit: Same as input  ParamDataTypeStr=Inherit: Same as input
  Ptrm1 : Sum  Inputs=+-  SaturateOnIntegerOverflow=on  InputSameDT=on  OutDataTypeStr=Inherit: Same as first input
  Wbatt starts at SOC_batt_ref : Integrator  InitialCondition=Wbatt*SOC_batt_ref/100  LimitOutput=on  UpperSaturationLimit=1.2*Wbatt  LowerSaturationLimit=0
  Wbatt [%] : Outport
  DeltaWbatt in [Ws] : Outport  Port=2
  wires:
  Wbatt starts at SOC_batt_ref/1 -> Gain3/1, Ptrm1/1
  Gain3/1 -> Wbatt [%]/1
  Constant/1 -> Ptrm1/2
  Ptrm1/1 -> DeltaWbatt in [Ws]/1
  "Pcharge "/1 -> Wbatt starts at SOC_batt_ref/1

== system Parallel_R2017b/EM (El.machine)/Subsystem ==
  T : Inport
  w : Inport  Port=2
  Abs2 : Abs  SaturateOnIntegerOverflow=on
  Constant : Constant  Value=eps
  EM torque1 : Product  Inputs=/*  SaturateOnIntegerOverflow=on  InputSameDT=on  OutDataTypeStr=Inherit: Same as first input
  T*w_ice : Product  Inputs=**  SaturateOnIntegerOverflow=on  InputSameDT=on  OutDataTypeStr=Inherit: Same as first input
  maxP : Saturate  UpperLimit=Pmax  LowerLimit=-Pmax
  maxT : Saturate  UpperLimit=Tmax  LowerLimit=-Tmax
  not div by 0 : Sum  SaturateOnIntegerOverflow=on  InputSameDT=on  OutDataTypeStr=Inherit: Same as first input
  Tlim : Outport
  wires:
  w/1 -> Abs2/1
  T/1 -> T*w_ice/2
  T*w_ice/1 -> maxP/1
  maxP/1 -> EM torque1/2
  maxT/1 -> Tlim/1
  EM torque1/1 -> maxT/1
  Constant/1 -> not div by 0/1
  not div by 0/1 -> EM torque1/1
  Abs2/1 -> T*w_ice/1, not div by 0/2

== system Parallel_R2017b/EM (El.machine)/wt (EM) ==
  x : Inport
  y : Inport  Port=2
  Mux : Mux  Inputs=2
  sfunxy : S-Function  DisableCoverage=on  FunctionName=sfunxy  Parameters=[xmin xmax ymin ymax], st  SFunctionDeploymentMode=off  EnableBusSupport=off
  wires:
  y/1 -> Mux/2
  x/1 -> Mux/1
  Mux/1 -> sfunxy/1

== system Parallel_R2017b/ICE-model/FuelPower ==
  Rows : Inport
  Cols : Inport  Port=2
  Look-Up Table (2-D) : Lookup2D  RowIndex=x  ColumnIndex=y  Table=t  SaturateOnIntegerOverflow=on  InputSameDT=on
  Out1 : Outport
  wires:
  Look-Up Table (2-D)/1 -> Out1/1
  Cols/1 -> Look-Up Table (2-D)/2
  Rows/1 -> Look-Up Table (2-D)/1

== system Parallel_R2017b/ICE-model/Generator of conventional vehicle ==
  ICE speed : Inport
  ICE on/off : Inport  Port=2
  Constant : Constant  Value=Paux
  Constant1 : Constant  Value=(1-Hybrid)
  Generator Efficiency : Constant  Value=0.5
  Generator Mech Power : Product  Inputs=/*  SaturateOnIntegerOverflow=on  InputSameDT=on  OutDataTypeStr=Inherit: Same as first input
  Generator Mech Torque : Product  Inputs=/**  SaturateOnIntegerOverflow=on  InputSameDT=on  OutDataTypeStr=Inherit: Same as first input
  Generator El Power : Product  Inputs=**  SaturateOnIntegerOverflow=on  InputSameDT=on  OutDataTypeStr=Inherit: Same as first input
  Generator torque : Outport
  wires:
  Constant/1 -> Generator El Power/2
  Generator El Power/1 -> Generator Mech Power/2
  Generator Efficiency/1 -> Generator Mech Power/1
  Generator Mech Power/1 -> Generator Mech Torque/2
  ICE speed/1 -> Generator Mech Torque/1
  ICE on/off/1 -> Generator El Power/1
  Generator Mech Torque/1 -> Generator torque/1
  Constant1/1 -> Generator Mech Torque/3

== system Parallel_R2017b/ICE-model/ICE efficiency ==
  Rows : Inport
  Cols : Inport  Port=2
  Look-Up Table (2-D) : Lookup2D  RowIndex=x  ColumnIndex=y  Table=t  SaturateOnIntegerOverflow=on  InputSameDT=on
  Out1 : Outport
  wires:
  Look-Up Table (2-D)/1 -> Out1/1
  Cols/1 -> Look-Up Table (2-D)/2
  Rows/1 -> Look-Up Table (2-D)/1

== system Parallel_R2017b/ICE-model/Medelvärde ==
  note: Denna del "mäter" tiden då motorn
      | är till, d.v.s. då verkningsgraden är
      | större än 1 %. Om den är 5 % antas
      | motorn stå still.
  In : Inport
  Integral : Integrator
  Integral1 : Integrator  InitialCondition=4  LimitOutput=on  LowerSaturationLimit=1
  Medelv : Product  Inputs=*/  SaturateOnIntegerOverflow=on  InputSameDT=on  OutDataTypeStr=Inherit: Same as first input
  Medelv1 : Product  Inputs=**  SaturateOnIntegerOverflow=on  InputSameDT=on  OutDataTypeStr=Inherit: Same as first input
  Mux : Mux  Inputs=2
  Relay : Relay  OnSwitchValue=0.05  OffSwitchValue=0.04
  Scope : Scope
  "Inst, Ave" : Outport
  tag scope: EtaICEave=global
  wires:
  Mux/1 -> "Inst, Ave"/1
  Medelv/1 -> Mux/2, [EtaICEave], Scope/1
  Relay/1 -> Integral1/1, Medelv1/2
  In/1 -> Mux/1, Relay/1, Medelv1/1
  Integral/1 -> Medelv/1
  Integral1/1 -> Medelv/2
  Medelv1/1 -> Integral/1

== system Parallel_R2017b/ICE-model/wt (ICE) ==
  x : Inport
  y : Inport  Port=2
  Mux : Mux  Inputs=2
  sfunxy : S-Function  DisableCoverage=on  FunctionName=sfunxy  Parameters=[xmin xmax ymin ymax], st  SFunctionDeploymentMode=off  EnableBusSupport=off
  wires:
  y/1 -> Mux/2
  x/1 -> Mux/1
  Mux/1 -> sfunxy/1

== system Parallel_R2017b/Power flow control/Charge control ==
  SOC : Inport
  10% deviation gives 10 kW : Gain  Gain=ksoc  OutDataTypeStr=Inherit: Same as input  ParamDataTypeStr=Inherit: Same as input
  Abs : Abs  SaturateOnIntegerOverflow=on
  Limit (Conv. Vehicle Generator max 2 kW) : Saturate  UpperLimit=Pem_max  LowerLimit=-Pem_max*Hybrid
  Look-Up Table : Lookup  InputValues=[-15:5:15]  Table=ksoc*[-3 -0.5 -0.1 0 0.1 0.5 3]  SaturateOnIntegerOverflow=on
  Manual Switch : ManualSwitch
  Mux : Mux  Inputs=2
  Product : Product  SaturateOnIntegerOverflow=on  OutDataTypeStr=Inherit: Same as first input
  SOC* : Constant  Value=SOC_batt_ref
  Scope : Scope  NumInputPorts=2
  Sum1 : Sum  Inputs=-+  SaturateOnIntegerOverflow=on  InputSameDT=on  OutDataTypeStr=Inherit: Same as first input
  P charge * : Outport  InitialOutput=0
  wires:
  SOC*/1 -> Sum1/2
  Sum1/1 -> 10% deviation gives 10 kW/1, Look-Up Table/1, Abs/1
  SOC/1 -> Sum1/1
  Limit (Conv. Vehicle Generator max 2 kW)/1 -> P charge */1
  Look-Up Table/1 -> Product/1
  10% deviation gives 10 kW/1 -> Manual Switch/1, Mux/1
  Product/1 -> Manual Switch/2, Mux/2
  Manual Switch/1 -> Limit (Conv. Vehicle Generator max 2 kW)/1
  Mux/1 -> Scope/1
  Abs/1 -> Product/2, Scope/2

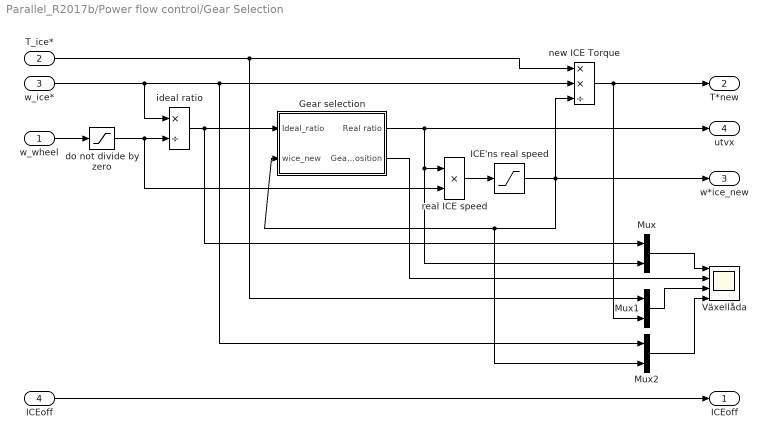
== system Parallel_R2017b/Power flow control/Gear Selection ==
  w_wheel : Inport
  T_ice* : Inport  Port=2
  w_ice* : Inport  Port=3
  ICEoff : Inport  Port=4
  Gear selection : Subsystem
  ICE'ns real speed : Saturate  UpperLimit=wice_max  LowerLimit=wice_min
  Mux : Mux  Inputs=2
  Mux1 : Mux  Inputs=2
  Mux2 : Mux  Inputs=2
  Växellåda : Scope  NumInputPorts=4
  do not divide by zero : Saturate  UpperLimit=inf  LowerLimit=1
  ideal ratio : Product  Inputs=*/  SaturateOnIntegerOverflow=on  InputSameDT=on  OutDataTypeStr=Inherit: Same as first input
  new ICE Torque : Product  Inputs=**/  SaturateOnIntegerOverflow=on  InputSameDT=on  OutDataTypeStr=Inherit: Same as first input
  real ICE speed : Product  Inputs=**  SaturateOnIntegerOverflow=on  InputSameDT=on  OutDataTypeStr=Inherit: Same as first input
  "ICEoff " : Outport
  T*new : Outport  Port=2
  w*ice_new : Outport  Port=3
  utvx : Outport  Port=4
  wires:
  w_ice*/1 -> ideal ratio/1, new ICE Torque/2, Mux2/1
  ideal ratio/1 -> Gear selection/1(Ideal_ratio), Mux/1
  T_ice*/1 -> new ICE Torque/1, Mux1/1
  do not divide by zero/1 -> ideal ratio/2, real ICE speed/2
  w_wheel/1 -> do not divide by zero/1
  Mux/1 -> Växellåda/1
  Mux1/1 -> Växellåda/3
  Mux2/1 -> Växellåda/4
  new ICE Torque/1 -> T*new/1, Mux1/2
  Gear selection/2(Gear position) -> Växellåda/2
  Gear selection/1(Real ratio) -> utvx/1, real ICE speed/1, Mux/2
  ICEoff/1 -> "ICEoff "/1
  real ICE speed/1 -> ICE'ns real speed/1
  ICE'ns real speed/1 -> new ICE Torque/3, w*ice_new/1, Mux2/2, Gear selection/2(wice_new)

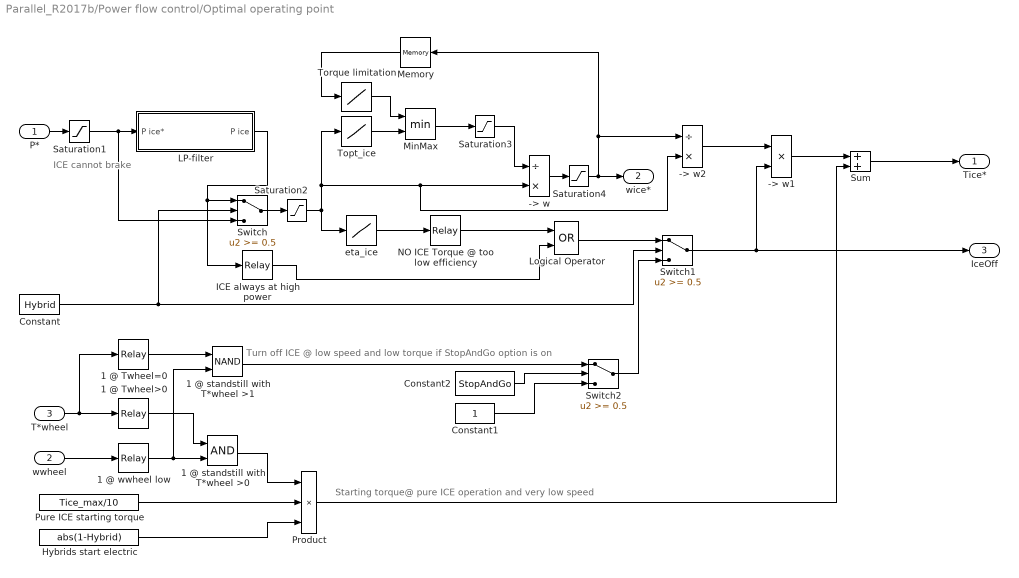
== system Parallel_R2017b/Power flow control/Optimal operating point ==
  note: ICE cannot
      | brake
  note: Starting torque@ pure ICE operation and very low speed
  note: Turn off ICE @ low speed and low torque if StopAndGo option is on
  P* : Inport
  wwheel : Inport  Port=2
  T*wheel : Inport  Port=3
  -> w : Product  Inputs=/*  SaturateOnIntegerOverflow=on  InputSameDT=on  OutDataTypeStr=Inherit: Same as first input
  -> w1 : Product  Inputs=**  SaturateOnIntegerOverflow=on  InputSameDT=on  OutDataTypeStr=Inherit: Same as first input
  -> w2 : Product  Inputs=/*  SaturateOnIntegerOverflow=on  InputSameDT=on  OutDataTypeStr=Inherit: Same as first input
  1 @ Twheel=0 : Relay  OnOutputValue=0  OffOutputValue=1
  1 @ Twheel>0 : Relay
  1 @ standstill with T*wheel >0 : Logic
  1 @ standstill with T*wheel >1 : Logic  Operator=NAND
  1 @ wwheel low : Relay  OnSwitchValue=1.1*wice_min/utvx_max  OffSwitchValue=0.9*wice_min/utvx_max  OnOutputValue=0  OffOutputValue=1
  Constant : Constant  Value=Hybrid
  Constant1 : Constant
  Constant2 : Constant  Value=StopAndGo
  Hybrids start electric : Constant  Value=abs(1-Hybrid)
  ICE always at high power : Relay  OnSwitchValue=Pice_max/2*1.1  OffSwitchValue=Pice_max/2*0.9
  LP-filter : Subsystem
  Logical Operator : Logic  Operator=OR  AllPortsSameDT=off
  Memory : Memory
  MinMax : MinMax  Inputs=2  SaturateOnIntegerOverflow=on  InputSameDT=on
  NO ICE Torque @ too low efficiency : Relay  OnSwitchValue=0.28  OffSwitchValue=0.25
  Product : Product  Inputs=3  SaturateOnIntegerOverflow=on  OutDataTypeStr=Inherit: Same as first input
  Pure ICE starting torque : Constant  Value=Tice_max/10
  Saturation1 : Saturate  UpperLimit=inf  LowerLimit=eps
  Saturation2 : Saturate  UpperLimit=Pice_max  LowerLimit=eps
  Saturation3 : Saturate  UpperLimit=inf  LowerLimit=eps
  Saturation4 : Saturate  UpperLimit=wice_max  LowerLimit=wice_min
  Sum : Sum  SaturateOnIntegerOverflow=on
  Switch : Switch  Threshold=0.5  SaturateOnIntegerOverflow=on  InputSameDT=on
  Switch1 : Switch  Threshold=0.5  SaturateOnIntegerOverflow=on  InputSameDT=on
  Switch2 : Switch  Threshold=0.5  SaturateOnIntegerOverflow=on  InputSameDT=on
  Topt_ice : Lookup  InputValues=PtoT(:,1)  Table=PtoT(:,2)  SaturateOnIntegerOverflow=on
  Torque limitation : Lookup  InputValues=Wice  Table=Tlim_ice  SaturateOnIntegerOverflow=on
  eta_ice : Lookup  InputValues=PtoT(:,1)  Table=PtoT(:,3)  SaturateOnIntegerOverflow=on
  Tice* : Outport  InitialOutput=0
  wice* : Outport  Port=2  InitialOutput=0
  IceOff : Outport  Port=3  InitialOutput=0
  wires:
  P*/1 -> Saturation1/1
  -> w/1 -> Saturation4/1
  eta_ice/1 -> NO ICE Torque @ too low efficiency/1
  Constant/1 -> Switch1/2, Switch/2
  Switch/1 -> Saturation2/1
  Switch1/1 -> -> w1/2, IceOff/1
  Saturation1/1 -> LP-filter/1(P ice*), Switch/3
  Saturation4/1 -> wice*/1, -> w2/1, Memory/1
  Saturation2/1 -> Topt_ice/1, -> w/2, -> w2/2, eta_ice/1
  -> w2/1 -> -> w1/1
  LP-filter/1(P ice) -> Switch/1, ICE always at high power/1
  NO ICE Torque @ too low efficiency/1 -> Logical Operator/1
  ICE always at high power/1 -> Logical Operator/2
  wwheel/1 -> 1 @ wwheel low/1
  T*wheel/1 -> 1 @ Twheel>0/1, 1 @ Twheel=0/1
  1 @ standstill with T*wheel >0/1 -> Product/1
  Pure ICE starting torque/1 -> Product/2
  Hybrids start electric/1 -> Product/3
  -> w1/1 -> Sum/1
  Sum/1 -> Tice*/1
  Product/1 -> Sum/2
  1 @ Twheel=0/1 -> 1 @ standstill with T*wheel >1/1
  1 @ wwheel low/1 -> 1 @ standstill with T*wheel >1/2, 1 @ standstill with T*wheel >0/2
  1 @ standstill with T*wheel >1/1 -> Switch2/1
  Constant1/1 -> Switch2/3
  Constant2/1 -> Switch2/2
  Switch2/1 -> Switch1/3
  Logical Operator/1 -> Switch1/1
  Torque limitation/1 -> MinMax/1
  Topt_ice/1 -> MinMax/2
  MinMax/1 -> Saturation3/1
  Memory/1 -> Torque limitation/1
  Saturation3/1 -> -> w/1
  1 @ Twheel>0/1 -> 1 @ standstill with T*wheel >0/1

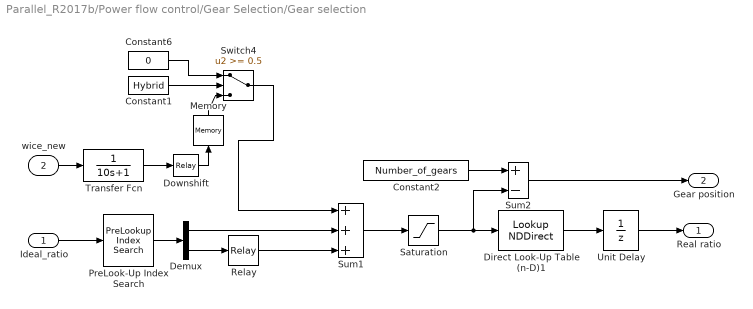
== system Parallel_R2017b/Power flow control/Gear Selection/Gear selection ==
  Ideal_ratio : Inport
  wice_new : Inport  Port=2
  Constant1 : Constant  Value=Hybrid
  Constant2 : Constant  Value=Number_of_gears
  Constant6 : Constant  Value=0
  Demux : Demux  Outputs=2
  Direct Look-Up Table (n-D)1 : LookupNDDirect  NumberOfTableDimensions=1  Table=Utvx_vect
  Downshift : Relay  OnSwitchValue=0.85*wice_max  OffSwitchValue=0.40*wice_max  OnOutputValue=0  OffOutputValue=Speedy
  Memory : Memory
  PreLook-Up Index Search : simulink_need_slupdate/PreLookup Index Search  bpData=Utvx_vect  searchMode=Binary Search  cacheBpFlag=off  outputFlag=off  IndexDataType=uint32  extrapMode=Linear Extrapolation  rangeErrorMode=None
      settings: SourceProductName=Simulink  SourceProductBaseCode=SL
  Relay : Relay  OnSwitchValue=0.55  OffSwitchValue=0.45
  Saturation : Saturate  UpperLimit=Number_of_gears-1  LowerLimit=0
  Sum1 : Sum  Inputs=+++  SaturateOnIntegerOverflow=on
  Sum2 : Sum  Inputs=+-  SaturateOnIntegerOverflow=on
  Switch4 : Switch  Threshold=0.5  SaturateOnIntegerOverflow=on  InputSameDT=on
  Transfer Fcn : TransferFcn  Denominator=[10 1]
  Unit Delay : UnitDelay  InitialCondition=utvx_max
  Real ratio : Outport
  Gear position : Outport  Port=2
  wires:
  Ideal_ratio/1 -> PreLook-Up Index Search/1
  Constant1/1 -> Switch4/2
  Switch4/1 -> Sum1/1
  wice_new/1 -> Transfer Fcn/1
  Downshift/1 -> Memory/1
  Transfer Fcn/1 -> Downshift/1
  Memory/1 -> Switch4/3
  Constant6/1 -> Switch4/1
  PreLook-Up Index Search/1 -> Demux/1
  Demux/2 -> Relay/1
  Sum1/1 -> Saturation/1
  Relay/1 -> Sum1/3
  Demux/1 -> Sum1/2
  Direct Look-Up Table (n-D)1/1 -> Unit Delay/1
  Constant2/1 -> Sum2/1
  Sum2/1 -> Gear position/1
  Unit Delay/1 -> Real ratio/1
  Saturation/1 -> Sum2/2, Direct Look-Up Table (n-D)1/1

== system Parallel_R2017b/Power flow control/Optimal operating point/LP-filter ==
  P ice* : Inport
  Gain2 : Gain  Gain=1/(Tau_charge)  SaturateOnIntegerOverflow=on  OutDataTypeStr=Inherit: Same as input  ParamDataTypeStr=Inherit: Same as input
  Sum3 : Sum  Inputs=+-  SaturateOnIntegerOverflow=on  InputSameDT=on  OutDataTypeStr=Inherit: Same as first input
  Wbatt : Integrator  UpperSaturationLimit=Pice_max_parallel  LowerSaturationLimit=0
  P ice : Outport  InitialOutput=0
  wires:
  P ice*/1 -> Sum3/1
  Sum3/1 -> Gain2/1
  Gain2/1 -> Wbatt/1
  Wbatt/1 -> Sum3/2, P ice/1
